simulink library "vehicle_role_lib"  (Simulink 8.2)
settings: Solver=ode1  StartTime=0.0  StopTime=Inf  FixedStep=0.001  RelTol=1e-3
PostLoadFcn:
  | , if any(exist('dsrtsu_mdlpostloadfcn', 'file') == [2, 3, 6]), try dsrtsu_mdlpostloadfcn('Execute', bdroot); catch fprintf('Error in PostLoadFcn (dsrtsu_mdlpostloadfcn) for model "%s":\n %s\n', bdroot, lasterr); end, end,
settings Model: DSRTSU_INTERNAL_RTI_VER=450  DSRTSU_INTERNAL_RTI_TYPE=rti1401  DSRTSU_INTERNAL_RTIFPGA=40  Creator=rushk1  LastModifiedBy=rushk1

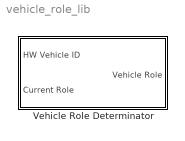
== system vehicle_role_lib ==
  Vehicle Role Determinator : Subsystem

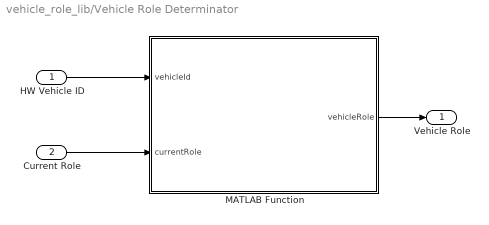
== system vehicle_role_lib/Vehicle Role Determinator ==
  HW Vehicle ID : Inport
  Current Role : Inport  Port=2
  MATLAB Function : MATLAB Function  TreatAsAtomicUnit=on
  Vehicle Role : Outport
  wires:
  HW Vehicle ID/1 -> MATLAB Function/1(vehicleId)
  MATLAB Function/1(vehicleRole) -> Vehicle Role/1
  Current Role/1 -> MATLAB Function/2(currentRole)

== matlab function Vehicle Role Determinator/MATLAB Function ==
  data: vehicleId input double; vehicleRole output double; currentRole input double
function vehicleRole = fcn(vehicleId, currentRole)
% Setup the map object
roleSet = [2, 3, 1, 0, 0];
if (currentRole == VehicleRoleEnum.ERROR)
    vehicleRole = VehicleRoleEnum(roleSet(vehicleId - 95));
else
    vehicleRole = currentRole;
end
